simulink model "World_01_Base_Map_cs"  (R2019a)
settings: Solver=FixedStepDiscrete  StartTime=0.0  StopTime=40  FixedStep=1/300  RelTol=1e-3
PreLoadFcn:
  | mbxruntime.callbacks.PreLoadFcn(bdroot);
  | check_NUTS_defined
  | model_closed = 0;
  | assignin('base',['model_closed_' bdroot],false);
PostLoadFcn:
  | mbxruntime.callbacks.PostLoadFcn(bdroot);
InitFcn:
  | mbxruntime.callbacks.InitFcn(bdroot);
StartFcn:
  | mbxruntime.callbacks.StartFcn(bdroot);
StopFcn:
  | mbxruntime.callbacks.StopFcn(bdroot);;
  | 
model workspace: external: MAT-File .\Base_Map_Closed_cs_hws.mat (data not in the file)
undefined symbols (not defined in the file): AngularVelocity, Clock_, Data, Data_SL_Info, DiscIntNeverNeededParam, Encoding, Encoding_SL_Info, Header, Height, InitImageOutputDir, LinearAcceleration, mbxruntime, Orientation, Pose, Poses, Poses_SL_Info, Position, Step, tabledata, Twist, Width
libraries: robotlib x26, simulink_extras x22, simulink x10, PreScanSimulinkLibrary x4, dspindex x4, sharedtransform x3, robotcorelib x2, visionconversions x2, visionsinks x2
(part 1 of 7)
CloseFcn:
  | mbxruntime.callbacks.CloseFcn(bdroot);
  | evalin('base',['clear model_closed_' bdroot]);
  | model_closed = 1;
settings Model: Creator=PRESCAN  LastModifiedBy=adeye
settings DataIOCC: LimitDataPoints=on  SaveFormat=Array  SignalLoggingSaveFormat=ModelDataLogs  ReturnWorkspaceOutputs=off
settings OptimizationCC: DefaultParameterBehavior=Inlined  ExpressionDepthLimit=2147483647  InitFltsAndDblsToZero=on  LifeSpan=inf
settings DebuggingCC: SaveWithParameterizedLinksMsg=none  UnderspecifiedInitializationDetection=Classic  MergeDetectMultiDrivingBlocksExec=none  SignalResolutionControl=TryResolveAllWithWarning  MultiTaskDSMMsg=warning  MultiTaskCondExecSysMsg=none  FcnCallInpInsideContextMsg=warning  StateNameClashWarn=warning  SFUnexpectedBacktrackingDiag=warning  SFNoUnconditionalDefaultTransitionDiag=warning  SFExecutionAtInitializationDiag=none  ArithmeticOperatorsInVariantConditions=warning
settings HardwareCC: ProdBitPerPointer=32  ProdBitPerSizeT=32  ProdBitPerPtrDiffT=32  ProdLargestAtomicFloat=None  ProdIntDivRoundTo=Undefined  ProdEndianess=Unspecified  ProdWordSize=32  ProdHWDeviceType=32-bit Generic
settings ModelReferenceCC: UpdateModelReferenceTargets=IfOutOfDate  PropagateSignalLabelsOutOfModel=off
settings SFSimCC: SimUseLocalCustomCode=off  SimParseCustomCode=off
settings SFSimCC: SimCustomHeaderCode=|
  | #include "prescan.h"
  | #include "prescan_platform.h"
settings RTWCC: RTWUseLocalCustomCode=off
settings CodeAppCC: StateflowObjectComments=on
settings GRTTargetCC: TargetFcnLib=ansi_tfl_tmw.mat  TargetLangStandard=C89/C90 (ANSI)  GeneratePreprocessorConditionals=Disable all  CombineOutputUpdateFcns=off  GRTInterface=on
settings ConfigComp: CovMetricSettings=dw  CovHtmlReporting=on  CovSaveCumulativeToWorkspaceVar=on  CovSaveSingleToWorkspaceVar=on  CovExternalEMLEnable=off

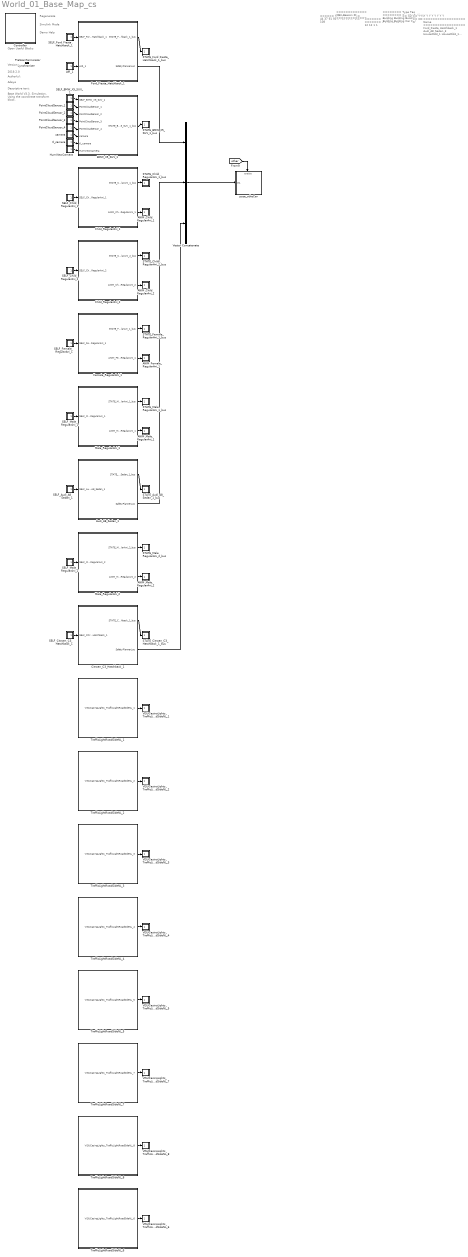
== system World_01_Base_Map_cs ==
  note: Regenerate
  note: Simulink Mode
  note: Open Useful Blocks
  note: 2019.2.0
  note: Version:
  note: Author(s):
  note: Adeye
  note: Descriptive text:
  note: Base World V3.3. Simulation,
      |
      |
      |
      | Using the coordinate transform
      | block.
  note: Demo Help
  note: ======
      | Num ID
      | ======
      | 44
      | 37
      | 91
      | 93
      | 94
      | 95
      | 96
      | 97
      | 102
      | 108
  note: =============
      | OBU-Beacon ID
      | =============
  note: =======
      | Type ID
      | =======
      | 1
      | 1
      | 12
      | 12
      | 12
      | 12
      | 12
      | 12
      | 1
      | 1
  note: ========
      | Type Tag
      | ========
      | Car
      | Car
      | Building
      | Building
      | Building
      | Building
      | Building
      | Building
      | Car
      | Car
  note: ==
      | SD
      | ==
      | Y
      | Y
      | Y
      | Y
      | Y
      | Y
      | Y
      | Y
      | Y
      | Y
  note: ==
      | CD
      | ==
      | N
      | N
      | N
      | N
      | N
      | N
      | N
      | N
      | N
      | N
  note: ==================
      | Name
      | ==================
      | Ford_Fiesta_Hatchback_1
      | Audi_A8_Sedan_3
      | HouseOld3_1
      | HouseOld4_1
      | HouseOld5_1
      | School_1
      | OfficeBrownFlat_1
      | OfficeBrownTall2_1
      | Audi_A8_Sedan_1
      | Citroen_C3_Hatchback_1
  AIR_1 : Subsystem  Tag=sensor/AIR  Priority=3  LoadFcn=load('PrescanAIRSensorData.mat');load('PrescanAIRSensorMessage.mat')  mask(PreScan Source Block: Actor Independent Receiver (AIR)){}
      mask help:
      | The Actor Information Receiver sensor provides a fast, simple and generic detection solution which is not tied up to a specific technology. The AIR detects the intersection point of the bounding box with the straight line from the sensor axis system to the middle of the bounding box.
      |
      | For more information, please click Help.
      settings: OpenFcn=open_system([gcb '/Sensor'],'mask')
      mask Help: eval('openHelp(413)')
      mask Display: image(imread('AIR.png'))
  ANIM_Child_RegularAni_1 : Subsystem  Tag=actuator/AnimationOutport  Priority=0  LoadFcn=load('PreScanAnimActuatorData.mat')  mask(PreScan Sink Block: State Animation){}
      mask help: The Human Animation port allows the human to walk, run or bend
      settings: OpenFcn=open_system([gcb '/Actuator'],'mask')
      mask Help: eval('openHelp(239)')
      mask Display: image(imread('HumanAnimated.jpg'))
  ANIM_Child_RegularAni_2 : Subsystem  Tag=actuator/AnimationOutport  Priority=0  LoadFcn=load('PreScanAnimActuatorData.mat')  mask(PreScan Sink Block: State Animation){}
      mask help: The Human Animation port allows the human to walk, run or bend
      settings: OpenFcn=open_system([gcb '/Actuator'],'mask')
      mask Help: eval('openHelp(239)')
      mask Display: image(imread('HumanAnimated.jpg'))
  ANIM_Female_RegularAni_1 : Subsystem  Tag=actuator/AnimationOutport  Priority=0  LoadFcn=load('PreScanAnimActuatorData.mat')  mask(PreScan Sink Block: State Animation){}
      mask help: The Human Animation port allows the human to walk, run or bend
      settings: OpenFcn=open_system([gcb '/Actuator'],'mask')
      mask Help: eval('openHelp(239)')
      mask Display: image(imread('HumanAnimated.jpg'))
  ANIM_Male_RegularAni_1 : Subsystem  Tag=actuator/AnimationOutport  Priority=0  LoadFcn=load('PreScanAnimActuatorData.mat')  mask(PreScan Sink Block: State Animation){}
      mask help: The Human Animation port allows the human to walk, run or bend
      settings: OpenFcn=open_system([gcb '/Actuator'],'mask')
      mask Help: eval('openHelp(239)')
      mask Display: image(imread('HumanAnimated.jpg'))
  ANIM_Male_RegularAni_2 : Subsystem  Tag=actuator/AnimationOutport  Priority=0  LoadFcn=load('PreScanAnimActuatorData.mat')  mask(PreScan Sink Block: State Animation){}
      mask help: The Human Animation port allows the human to walk, run or bend
      settings: OpenFcn=open_system([gcb '/Actuator'],'mask')
      mask Help: eval('openHelp(239)')
      mask Display: image(imread('HumanAnimated.jpg'))
  Audi_A8_Sedan_1 : Subsystem  Tag=WorldObjectSubSystem  InitFcn=UniqueId = '18645';
      mask init:
      | modelPath = GenericModelHelper.getGenericModelFilePath('ModelDepo','Vehicles\Audi_A8\Audi_A8.pgmb','e33fe1ddcf3e8ae97caccbc8f2fa74ac');imagePath = GenericModelHelper.getCompilationPicture(modelPath, 'Audi_A8_HighPoly.png');
      mask Display: image(imread(imagePath));color('white');text(0, 0, ' ID=102\n')
  BMW_X5_SUV_1 : Subsystem  Tag=WorldObjectSubSystem  InitFcn=UniqueId = '9040';
      mask init:
      | modelPath = GenericModelHelper.getGenericModelFilePath('ModelDepo','Vehicles\BMW_X5\BMW_X5.pgmb','bfeb1c11467705ab888b3011684c848b');imagePath = GenericModelHelper.getCompilationPicture(modelPath, 'BMW_X5_HighPoly.png');
      mask Display: image(imread(imagePath));color('white');text(0, 0, ' ID=55\n')
  Child_RegularAni_1 : Subsystem  Tag=WorldObjectSubSystem  InitFcn=UniqueId = '18395';
      mask init:
      | imagePath=which('Child_RegularAni.jpg');
      mask Display: image(imread(imagePath));color('white');text(0, 0, ' ID=112\n')
  Child_RegularAni_2 : Subsystem  Tag=WorldObjectSubSystem  InitFcn=UniqueId = '18628';
      mask init:
      | imagePath=which('Child_RegularAni.jpg');
      mask Display: image(imread(imagePath));color('white');text(0, 0, ' ID=111\n')
  Citroen_C3_Hatchback_1 : Subsystem  Tag=WorldObjectSubSystem  InitFcn=UniqueId = '18857';
      mask init:
      | modelPath = GenericModelHelper.getGenericModelFilePath('ModelDepo','Vehicles\Citroen_C3\Citroen_C3.pgmb','e804ced06d50dbfc6a2202ab3ad01b0c');imagePath = GenericModelHelper.getCompilationPicture(modelPath, 'Citroen_C3_HighPoly.png');
      mask Display: image(imread(imagePath));color('white');text(0, 0, ' ID=108\n')
  Controller : Subsystem  Description=8A3CD2955739A82C886C20AE3E253D78460D53180EE2C1B14CC08DF75A70BE77  Priority=-1  LoadFcn=load PreScanControllerData  mask(PreScan Simulation Controller){prescanversion='2019.2.0', ModelReferencing=off, TimeStep=1/300, ControlMode=0, PreScanExecutionMode=on, ControllerCount=0, ControllerIndex=0, ControllerOptions=''}
      mask prompts: prescanversion "PreScan Version"; ModelReferencing "Use Model Referencing"; TimeStep "Upload Period [s]"; ControlMode "Control Mode"; PreScanExecutionMode "Execution Mode"; ControllerCount "Controller Count"; ControllerIndex "Controller Index"; ControllerOptions "Controller Options"
      mask help:
      | Please do not remove this block from the compilation sheet,
      | as it connects the model to the PreScan environment.
      mask init:
      | model = bdroot(gcb);
      | ExperimentFile = mbxruntime.findExperimentFile(model,true); %relative path
      | 
      | [d1, d2, d3, prescandata] = prescan_Settings();
      | ModelDepo = fullfile(prescandata,'ModelDepo'); 
      | 
      | RTmode = mbxruntime.getRTMode(model);
      | 
      | SimulationMode = get_param(bdroot,'SimulationMode');
      | if strcmp(SimulationMode, 'rapid-accelerator')
      |     SimulationMode = 'external';
      | end
      | TargetName = get_param(bdroot,'SystemTargetFile');
      settings: ModelCloseFcn=assignin('base',['model_closed_' bdroot],true);
      mask Help: eval('openHelp(812)')
      mask Display: image(imread('prescanlogo.ico'))
  Female_RegularAni_1 : Subsystem  Tag=WorldObjectSubSystem  InitFcn=UniqueId = '18631';
      mask init:
      | imagePath=which('Female_RegularAni.jpg');
      mask Display: image(imread(imagePath));color('white');text(0, 0, ' ID=113\n')
  Ford_Fiesta_Hatchback_1 : Subsystem  Tag=WorldObjectSubSystem  InitFcn=UniqueId = '4876';
      mask init:
      | modelPath = GenericModelHelper.getGenericModelFilePath('ModelDepo','Vehicles\Ford_Fiesta\Ford_Fiesta.pgmb','fe2c7a73e0a60cba76689b71cd1bb76a');imagePath = GenericModelHelper.getCompilationPicture(modelPath, 'Ford_Fiesta_HighPoly.png');
      mask Display: image(imread(imagePath));color('white');text(0, 0, ' ID=44\n')
  HumViewCamera : Subsystem  Tag=sensor/Camera/CameraSensor  Priority=3  mask(PreScan Source Block: Camera Sensor){}
      mask help: The Camera Sensor provides a color or monochrome image.
      settings: OpenFcn=open_system([gcb '/Sensor'],'mask')
      mask Help: eval('openHelp(457)')
      mask Display: image(imread('CameraSensor.png'))
  Male_RegularAni_1 : Subsystem  Tag=WorldObjectSubSystem  InitFcn=UniqueId = '18634';
      mask init:
      | imagePath=which('Male_RegularAni.jpg');
      mask Display: image(imread(imagePath));color('white');text(0, 0, ' ID=114\n')
  Male_RegularAni_2 : Subsystem  Tag=WorldObjectSubSystem  InitFcn=UniqueId = '18853';
      mask init:
      | imagePath=which('Male_RegularAni.jpg');
      mask Display: image(imread(imagePath));color('white');text(0, 0, ' ID=107\n')
  PointCloudSensor_1 : Subsystem  Tag=sensor/PointCloudInport  Priority=3  mask(PreScan Source Block: Point Cloud Sensor){}
      mask help: The Point Cloud Sensor provides XYZ positions relative to the sensor
      settings: OpenFcn=open_system([gcb '/Sensor'],'mask')
      mask Help: eval('openHelp(6400)')
      mask Display: image(imread('PointCloudSensorSL.png'))
  PointCloudSensor_2 : Subsystem  Tag=sensor/PointCloudInport  Priority=3  mask(PreScan Source Block: Point Cloud Sensor){}
      mask help: The Point Cloud Sensor provides XYZ positions relative to the sensor
      settings: OpenFcn=open_system([gcb '/Sensor'],'mask')
      mask Help: eval('openHelp(6400)')
      mask Display: image(imread('PointCloudSensorSL.png'))
  PointCloudSensor_3 : Subsystem  Tag=sensor/PointCloudInport  Priority=3  mask(PreScan Source Block: Point Cloud Sensor){}
      mask help: The Point Cloud Sensor provides XYZ positions relative to the sensor
      settings: OpenFcn=open_system([gcb '/Sensor'],'mask')
      mask Help: eval('openHelp(6400)')
      mask Display: image(imread('PointCloudSensorSL.png'))
  PointCloudSensor_4 : Subsystem  Tag=sensor/PointCloudInport  Priority=3  mask(PreScan Source Block: Point Cloud Sensor){}
      mask help: The Point Cloud Sensor provides XYZ positions relative to the sensor
      settings: OpenFcn=open_system([gcb '/Sensor'],'mask')
      mask Help: eval('openHelp(6400)')
      mask Display: image(imread('PointCloudSensorSL.png'))
  PreScanTerminator : Subsystem  Tag=PreScanTerminator  Priority=999  LoadFcn=load PrescanTerminatorData  mask(PreScan Simulation Terminator){TimeStep=1/300}
      mask prompts: TimeStep "Upload Period [s]"
      mask help:
      | Please do not remove this block from the compilation sheet as it
      | connects the model to the PreScan environment.
      mask Help: eval('openHelp(812)')
      mask Display: image(imread('prescanlogo.ico'))
  SELF_Audi_A8_Sedan_1 : Subsystem  Tag=sensor/SelfPort  Priority=3  LoadFcn=load('PreScanSelfSensorData.mat')  mask(PreScan Source Block: SELF){}
      mask help:
      | The SELF port shows (state) information of the actor itself. The outputs are position in the experiment's axis system and the GPS coordinates, and the object's absolute velocity and compass heading.
      |
      | For more information, please click Help.
      settings: OpenFcn=open_system([gcb '/Sensor'],'mask')
      mask Help: eval('openHelp(462)')
      mask Display: image(imread('GPS.png'))
  SELF_BMW_X5_SUV_1 : Subsystem  Tag=sensor/SelfPort  Priority=3  LoadFcn=load('PreScanSelfSensorData.mat')  mask(PreScan Source Block: SELF){}
      mask help:
      | The SELF port shows (state) information of the actor itself. The outputs are position in the experiment's axis system and the GPS coordinates, and the object's absolute velocity and compass heading.
      |
      | For more information, please click Help.
      settings: OpenFcn=open_system([gcb '/Sensor'],'mask')
      mask Help: eval('openHelp(462)')
      mask Display: image(imread('GPS.png'))
  SELF_Child_RegularAni_1 : Subsystem  Tag=sensor/SelfPort  Priority=3  LoadFcn=load('PreScanSelfSensorData.mat')  mask(PreScan Source Block: SELF){}
      mask help:
      | The SELF port shows (state) information of the actor itself. The outputs are position in the experiment's axis system and the GPS coordinates, and the object's absolute velocity and compass heading.
      |
      | For more information, please click Help.
      settings: OpenFcn=open_system([gcb '/Sensor'],'mask')
      mask Help: eval('openHelp(462)')
      mask Display: image(imread('GPS.png'))
  SELF_Child_RegularAni_2 : Subsystem  Tag=sensor/SelfPort  Priority=3  LoadFcn=load('PreScanSelfSensorData.mat')  mask(PreScan Source Block: SELF){}
      mask help:
      | The SELF port shows (state) information of the actor itself. The outputs are position in the experiment's axis system and the GPS coordinates, and the object's absolute velocity and compass heading.
      |
      | For more information, please click Help.
      settings: OpenFcn=open_system([gcb '/Sensor'],'mask')
      mask Help: eval('openHelp(462)')
      mask Display: image(imread('GPS.png'))
  SELF_Citroen_C3_Hatchback_1 : Subsystem  Tag=sensor/SelfPort  Priority=3  LoadFcn=load('PreScanSelfSensorData.mat')  mask(PreScan Source Block: SELF){}
      mask help:
      | The SELF port shows (state) information of the actor itself. The outputs are position in the experiment's axis system and the GPS coordinates, and the object's absolute velocity and compass heading.
      |
      | For more information, please click Help.
      settings: OpenFcn=open_system([gcb '/Sensor'],'mask')
      mask Help: eval('openHelp(462)')
      mask Display: image(imread('GPS.png'))
  SELF_Female_RegularAni_1 : Subsystem  Tag=sensor/SelfPort  Priority=3  LoadFcn=load('PreScanSelfSensorData.mat')  mask(PreScan Source Block: SELF){}
      mask help:
      | The SELF port shows (state) information of the actor itself. The outputs are position in the experiment's axis system and the GPS coordinates, and the object's absolute velocity and compass heading.
      |
      | For more information, please click Help.
      settings: OpenFcn=open_system([gcb '/Sensor'],'mask')
      mask Help: eval('openHelp(462)')
      mask Display: image(imread('GPS.png'))
  SELF_Ford_Fiesta_Hatchback_1 : Subsystem  Tag=sensor/SelfPort  Priority=3  LoadFcn=load('PreScanSelfSensorData.mat')  mask(PreScan Source Block: SELF){}
      mask help:
      | The SELF port shows (state) information of the actor itself. The outputs are position in the experiment's axis system and the GPS coordinates, and the object's absolute velocity and compass heading.
      |
      | For more information, please click Help.
      settings: OpenFcn=open_system([gcb '/Sensor'],'mask')
      mask Help: eval('openHelp(462)')
      mask Display: image(imread('GPS.png'))
  SELF_Male_RegularAni_1 : Subsystem  Tag=sensor/SelfPort  Priority=3  LoadFcn=load('PreScanSelfSensorData.mat')  mask(PreScan Source Block: SELF){}
      mask help:
      | The SELF port shows (state) information of the actor itself. The outputs are position in the experiment's axis system and the GPS coordinates, and the object's absolute velocity and compass heading.
      |
      | For more information, please click Help.
      settings: OpenFcn=open_system([gcb '/Sensor'],'mask')
      mask Help: eval('openHelp(462)')
      mask Display: image(imread('GPS.png'))
  SELF_Male_RegularAni_2 : Subsystem  Tag=sensor/SelfPort  Priority=3  LoadFcn=load('PreScanSelfSensorData.mat')  mask(PreScan Source Block: SELF){}
      mask help:
      | The SELF port shows (state) information of the actor itself. The outputs are position in the experiment's axis system and the GPS coordinates, and the object's absolute velocity and compass heading.
      |
      | For more information, please click Help.
      settings: OpenFcn=open_system([gcb '/Sensor'],'mask')
      mask Help: eval('openHelp(462)')
      mask Display: image(imread('GPS.png'))
  STATE_Audi_A8_Sedan_1_bus : Subsystem  Tag=actuator/StatePort  Priority=0  LoadFcn=load('PreScanStateActuatorData.mat')  mask(PreScan Sink Block: State){}
      mask help:
      | The Actor State contains a vector signal of size (9x1), containing the following signals:
      |
      | -  Position    	(x,y,z)             	[m]
      | -  Velocity    	(vx,vy,vz)         	[m/s]
      | -  Angles       	(Roll, Pitch, Yaw)	[rad]
      |
      | The Actor state is defined in the global axis system.
      | The state is superponed on the Initial position defined in the GUI.
      |
      | For more information, please click Help.
      settings: OpenFcn=open_system([gcb '/Actuator'],'mask')
      mask Help: eval('openHelp(222)')
      mask Display: image(imread('State.png'))
  STATE_BMW_X5_SUV_1_bus : Subsystem  Tag=actuator/StatePort  Priority=0  LoadFcn=load('PreScanStateActuatorData.mat')  mask(PreScan Sink Block: State){}
      mask help:
      | The Actor State contains a vector signal of size (9x1), containing the following signals:
      |
      | -  Position    	(x,y,z)             	[m]
      | -  Velocity    	(vx,vy,vz)         	[m/s]
      | -  Angles       	(Roll, Pitch, Yaw)	[rad]
      |
      | The Actor state is defined in the global axis system.
      | The state is superponed on the Initial position defined in the GUI.
      |
      | For more information, please click Help.
      settings: OpenFcn=open_system([gcb '/Actuator'],'mask')
      mask Help: eval('openHelp(222)')
      mask Display: image(imread('State.png'))
  STATE_Child_RegularAni_1_bus : Subsystem  Tag=actuator/StatePort  Priority=0  LoadFcn=load('PreScanStateActuatorData.mat')  mask(PreScan Sink Block: State){}
      mask help:
      | The Actor State contains a vector signal of size (9x1), containing the following signals:
      |
      | -  Position    	(x,y,z)             	[m]
      | -  Velocity    	(vx,vy,vz)         	[m/s]
      | -  Angles       	(Roll, Pitch, Yaw)	[rad]
      |
      | The Actor state is defined in the global axis system.
      | The state is superponed on the Initial position defined in the GUI.
      |
      | For more information, please click Help.
      settings: OpenFcn=open_system([gcb '/Actuator'],'mask')
      mask Help: eval('openHelp(222)')
      mask Display: image(imread('State.png'))
  STATE_Child_RegularAni_2_bus : Subsystem  Tag=actuator/StatePort  Priority=0  LoadFcn=load('PreScanStateActuatorData.mat')  mask(PreScan Sink Block: State){}
      mask help:
      | The Actor State contains a vector signal of size (9x1), containing the following signals:
      |
      | -  Position    	(x,y,z)             	[m]
      | -  Velocity    	(vx,vy,vz)         	[m/s]
      | -  Angles       	(Roll, Pitch, Yaw)	[rad]
      |
      | The Actor state is defined in the global axis system.
      | The state is superponed on the Initial position defined in the GUI.
      |
      | For more information, please click Help.
      settings: OpenFcn=open_system([gcb '/Actuator'],'mask')
      mask Help: eval('openHelp(222)')
      mask Display: image(imread('State.png'))
  STATE_Citroen_C3_Hatchback_1_bus : Subsystem  Tag=actuator/StatePort  Priority=0  LoadFcn=load('PreScanStateActuatorData.mat')  mask(PreScan Sink Block: State){}
      mask help:
      | The Actor State contains a vector signal of size (9x1), containing the following signals:
      |
      | -  Position    	(x,y,z)             	[m]
      | -  Velocity    	(vx,vy,vz)         	[m/s]
      | -  Angles       	(Roll, Pitch, Yaw)	[rad]
      |
      | The Actor state is defined in the global axis system.
      | The state is superponed on the Initial position defined in the GUI.
      |
      | For more information, please click Help.
      settings: OpenFcn=open_system([gcb '/Actuator'],'mask')
      mask Help: eval('openHelp(222)')
      mask Display: image(imread('State.png'))
  STATE_Female_RegularAni_1_bus : Subsystem  Tag=actuator/StatePort  Priority=0  LoadFcn=load('PreScanStateActuatorData.mat')  mask(PreScan Sink Block: State){}
      mask help:
      | The Actor State contains a vector signal of size (9x1), containing the following signals:
      |
      | -  Position    	(x,y,z)             	[m]
      | -  Velocity    	(vx,vy,vz)         	[m/s]
      | -  Angles       	(Roll, Pitch, Yaw)	[rad]
      |
      | The Actor state is defined in the global axis system.
      | The state is superponed on the Initial position defined in the GUI.
      |
      | For more information, please click Help.
      settings: OpenFcn=open_system([gcb '/Actuator'],'mask')
      mask Help: eval('openHelp(222)')
      mask Display: image(imread('State.png'))
  STATE_Ford_Fiesta_Hatchback_1_bus : Subsystem  Tag=actuator/StatePort  Priority=0  LoadFcn=load('PreScanStateActuatorData.mat')  mask(PreScan Sink Block: State){}
      mask help:
      | The Actor State contains a vector signal of size (9x1), containing the following signals:
      |
      | -  Position    	(x,y,z)             	[m]
      | -  Velocity    	(vx,vy,vz)         	[m/s]
      | -  Angles       	(Roll, Pitch, Yaw)	[rad]
      |
      | The Actor state is defined in the global axis system.
      | The state is superponed on the Initial position defined in the GUI.
      |
      | For more information, please click Help.
      settings: OpenFcn=open_system([gcb '/Actuator'],'mask')
      mask Help: eval('openHelp(222)')
      mask Display: image(imread('State.png'))
  STATE_Male_RegularAni_1_bus : Subsystem  Tag=actuator/StatePort  Priority=0  LoadFcn=load('PreScanStateActuatorData.mat')  mask(PreScan Sink Block: State){}
      mask help:
      | The Actor State contains a vector signal of size (9x1), containing the following signals:
      |
      | -  Position    	(x,y,z)             	[m]
      | -  Velocity    	(vx,vy,vz)         	[m/s]
      | -  Angles       	(Roll, Pitch, Yaw)	[rad]
      |
      | The Actor state is defined in the global axis system.
      | The state is superponed on the Initial position defined in the GUI.
      |
      | For more information, please click Help.
      settings: OpenFcn=open_system([gcb '/Actuator'],'mask')
      mask Help: eval('openHelp(222)')
      mask Display: image(imread('State.png'))
  STATE_Male_RegularAni_2_bus : Subsystem  Tag=actuator/StatePort  Priority=0  LoadFcn=load('PreScanStateActuatorData.mat')  mask(PreScan Sink Block: State){}
      mask help:
      | The Actor State contains a vector signal of size (9x1), containing the following signals:
      |
      | -  Position    	(x,y,z)             	[m]
      | -  Velocity    	(vx,vy,vz)         	[m/s]
      | -  Angles       	(Roll, Pitch, Yaw)	[rad]
      |
      | The Actor state is defined in the global axis system.
      | The state is superponed on the Initial position defined in the GUI.
      |
      | For more information, please click Help.
      settings: OpenFcn=open_system([gcb '/Actuator'],'mask')
      mask Help: eval('openHelp(222)')
      mask Display: image(imread('State.png'))
  Synchronizer : Subsystem  Tag=PreScanSynchronizer  Priority=1  LoadFcn=load PrescanSynchronizeData  mask(PreScan Simulation Core Block){TimeStep=1/300}
      mask prompts: TimeStep "Timestep [s]"
      mask help:
      | Please do not remove this block from the PreScan compilation sheet,
      | as it contains essential configuration parameters for a PreScan simulation.
      settings: DeleteFcn=PreScanBlockDeleteFcn;
      mask Display: image(imread('prescanlogo.ico'))
  TrafficLightRoadSideNL_1 : Subsystem  Tag=WorldObjectSubSystem  InitFcn=UniqueId = '646';
      mask init:
      | imagePath=which('TrafficLightRoadSideNL.jpg');
      mask Display: image(imread(imagePath));color('white');text(0, 0, ' ID=76\n')
  TrafficLightRoadSideNL_2 : Subsystem  Tag=WorldObjectSubSystem  InitFcn=UniqueId = '647';
      mask init:
      | imagePath=which('TrafficLightRoadSideNL.jpg');
      mask Display: image(imread(imagePath));color('white');text(0, 0, ' ID=77\n')
  TrafficLightRoadSideNL_3 : Subsystem  Tag=WorldObjectSubSystem  InitFcn=UniqueId = '649';
      mask init:
      | imagePath=which('TrafficLightRoadSideNL.jpg');
      mask Display: image(imread(imagePath));color('white');text(0, 0, ' ID=78\n')
  TrafficLightRoadSideNL_4 : Subsystem  Tag=WorldObjectSubSystem  InitFcn=UniqueId = '650';
      mask init:
      | imagePath=which('TrafficLightRoadSideNL.jpg');
      mask Display: image(imread(imagePath));color('white');text(0, 0, ' ID=79\n')
  TrafficLightRoadSideNL_5 : Subsystem  Tag=WorldObjectSubSystem  InitFcn=UniqueId = '651';
      mask init:
      | imagePath=which('TrafficLightRoadSideNL.jpg');
      mask Display: image(imread(imagePath));color('white');text(0, 0, ' ID=80\n')
  TrafficLightRoadSideNL_6 : Subsystem  Tag=WorldObjectSubSystem  InitFcn=UniqueId = '10446';
      mask init:
      | imagePath=which('TrafficLightRoadSideNL.jpg');
      mask Display: image(imread(imagePath));color('white');text(0, 0, ' ID=81\n')
  TrafficLightRoadSideNL_7 : Subsystem  Tag=WorldObjectSubSystem  InitFcn=UniqueId = '653';
      mask init:
      | imagePath=which('TrafficLightRoadSideNL.jpg');
      mask Display: image(imread(imagePath));color('white');text(0, 0, ' ID=82\n')
  TrafficLightRoadSideNL_8 : Subsystem  Tag=WorldObjectSubSystem  InitFcn=UniqueId = '654';
      mask init:
      | imagePath=which('TrafficLightRoadSideNL.jpg');
      mask Display: image(imread(imagePath));color('white');text(0, 0, ' ID=83\n')
  VISUCasingLights_TrafficLightRoadSideNL_1 : Subsystem  Tag=actuator/VisuCasingLights  Priority=0  mask(PreScan Sink Block: VisuTrafficLight){UniqueID=646, ColorsObjectQuery=, Colors=[]}
      mask prompts: UniqueID "Parent Unique Identifier"; ColorsObjectQuery "Query for Color Object"; Colors "Matrix of colors"
      mask help:
      | The VisuTrafficLight block provides a way to animate traffic lights: switch on and off individual lights.
      |
      | For more information, please click Help.
      settings: OpenFcn=open_system([gcb '/Actuator'],'mask')
      mask Help: eval('openHelp(731)')
      mask Display: image(imread('TrafficLightCasing.png'))
  VISUCasingLights_TrafficLightRoadSideNL_2 : Subsystem  Tag=actuator/VisuCasingLights  Priority=0  mask(PreScan Sink Block: VisuTrafficLight){UniqueID=647, ColorsObjectQuery=, Colors=[]}
      mask prompts: UniqueID "Parent Unique Identifier"; ColorsObjectQuery "Query for Color Object"; Colors "Matrix of colors"
      mask help:
      | The VisuTrafficLight block provides a way to animate traffic lights: switch on and off individual lights.
      |
      | For more information, please click Help.
      settings: OpenFcn=open_system([gcb '/Actuator'],'mask')
      mask Help: eval('openHelp(731)')
      mask Display: image(imread('TrafficLightCasing.png'))
  VISUCasingLights_TrafficLightRoadSideNL_3 : Subsystem  Tag=actuator/VisuCasingLights  Priority=0  mask(PreScan Sink Block: VisuTrafficLight){UniqueID=649, ColorsObjectQuery=, Colors=[]}
      mask prompts: UniqueID "Parent Unique Identifier"; ColorsObjectQuery "Query for Color Object"; Colors "Matrix of colors"
      mask help:
      | The VisuTrafficLight block provides a way to animate traffic lights: switch on and off individual lights.
      |
      | For more information, please click Help.
      settings: OpenFcn=open_system([gcb '/Actuator'],'mask')
      mask Help: eval('openHelp(731)')
      mask Display: image(imread('TrafficLightCasing.png'))
  VISUCasingLights_TrafficLightRoadSideNL_4 : Subsystem  Tag=actuator/VisuCasingLights  Priority=0  mask(PreScan Sink Block: VisuTrafficLight){UniqueID=650, ColorsObjectQuery=, Colors=[]}
      mask prompts: UniqueID "Parent Unique Identifier"; ColorsObjectQuery "Query for Color Object"; Colors "Matrix of colors"
      mask help:
      | The VisuTrafficLight block provides a way to animate traffic lights: switch on and off individual lights.
      |
      | For more information, please click Help.
      settings: OpenFcn=open_system([gcb '/Actuator'],'mask')
      mask Help: eval('openHelp(731)')
      mask Display: image(imread('TrafficLightCasing.png'))
  VISUCasingLights_TrafficLightRoadSideNL_5 : Subsystem  Tag=actuator/VisuCasingLights  Priority=0  mask(PreScan Sink Block: VisuTrafficLight){UniqueID=651, ColorsObjectQuery=, Colors=[]}
      mask prompts: UniqueID "Parent Unique Identifier"; ColorsObjectQuery "Query for Color Object"; Colors "Matrix of colors"
      mask help:
      | The VisuTrafficLight block provides a way to animate traffic lights: switch on and off individual lights.
      |
      | For more information, please click Help.
      settings: OpenFcn=open_system([gcb '/Actuator'],'mask')
      mask Help: eval('openHelp(731)')
      mask Display: image(imread('TrafficLightCasing.png'))
  VISUCasingLights_TrafficLightRoadSideNL_6 : Subsystem  Tag=actuator/VisuCasingLights  Priority=0  mask(PreScan Sink Block: VisuTrafficLight){UniqueID=10446, ColorsObjectQuery=, Colors=[]}
      mask prompts: UniqueID "Parent Unique Identifier"; ColorsObjectQuery "Query for Color Object"; Colors "Matrix of colors"
      mask help:
      | The VisuTrafficLight block provides a way to animate traffic lights: switch on and off individual lights.
      |
      | For more information, please click Help.
      settings: OpenFcn=open_system([gcb '/Actuator'],'mask')
      mask Help: eval('openHelp(731)')
      mask Display: image(imread('TrafficLightCasing.png'))
  VISUCasingLights_TrafficLightRoadSideNL_7 : Subsystem  Tag=actuator/VisuCasingLights  Priority=0  mask(PreScan Sink Block: VisuTrafficLight){UniqueID=653, ColorsObjectQuery=, Colors=[]}
      mask prompts: UniqueID "Parent Unique Identifier"; ColorsObjectQuery "Query for Color Object"; Colors "Matrix of colors"
      mask help:
      | The VisuTrafficLight block provides a way to animate traffic lights: switch on and off individual lights.
      |
      | For more information, please click Help.
      settings: OpenFcn=open_system([gcb '/Actuator'],'mask')
      mask Help: eval('openHelp(731)')
      mask Display: image(imread('TrafficLightCasing.png'))
  VISUCasingLights_TrafficLightRoadSideNL_8 : Subsystem  Tag=actuator/VisuCasingLights  Priority=0  mask(PreScan Sink Block: VisuTrafficLight){UniqueID=654, ColorsObjectQuery=, Colors=[]}
      mask prompts: UniqueID "Parent Unique Identifier"; ColorsObjectQuery "Query for Color Object"; Colors "Matrix of colors"
      mask help:
      | The VisuTrafficLight block provides a way to animate traffic lights: switch on and off individual lights.
      |
      | For more information, please click Help.
      settings: OpenFcn=open_system([gcb '/Actuator'],'mask')
      mask Help: eval('openHelp(731)')
      mask Display: image(imread('TrafficLightCasing.png'))
  Vector Concatenate : Concatenate  NumInputs=3
  camera : Subsystem  Tag=sensor/Camera/CameraSensor  Priority=3  mask(PreScan Source Block: Camera Sensor){}
      mask help: The Camera Sensor provides a color or monochrome image.
      settings: OpenFcn=open_system([gcb '/Sensor'],'mask')
      mask Help: eval('openHelp(457)')
      mask Display: image(imread('CameraSensor.png'))
  pose_otheCar : Subsystem
  tl_camera : Subsystem  Tag=sensor/Camera/CameraSensor  Priority=3  mask(PreScan Source Block: Camera Sensor){}
      mask help: The Camera Sensor provides a color or monochrome image.
      settings: OpenFcn=open_system([gcb '/Sensor'],'mask')
      mask Help: eval('openHelp(457)')
      mask Display: image(imread('CameraSensor.png'))
  wires:
  [other] -> pose_otheCar/Enable
  Vector Concatenate/1 -> pose_otheCar/1(In1)
  Ford_Fiesta_Hatchback_1/2(SafetyPlannerLoc) -> Vector Concatenate/1
  Audi_A8_Sedan_1/2(SafetyPlannerLoc) -> Vector Concatenate/2
  Citroen_C3_Hatchback_1/2(SafetyPlannerLoc) -> Vector Concatenate/3
  Ford_Fiesta_Hatchback_1/1(STATE_Ford_Fiesta_Hatchback_1_bus) -> STATE_Ford_Fiesta_Hatchback_1_bus/1(STATE_Ford_Fiesta_Hatchback_1_bus)
  SELF_Ford_Fiesta_Hatchback_1/1(SELF_Ford_Fiesta_Hatchback_1) -> Ford_Fiesta_Hatchback_1/1(SELF_Ford_Fiesta_Hatchback_1)
  AIR_1/1(AIR_1) -> Ford_Fiesta_Hatchback_1/2(AIR_1)
  BMW_X5_SUV_1/1(STATE_BMW_X5_SUV_1_bus) -> STATE_BMW_X5_SUV_1_bus/1(STATE_BMW_X5_SUV_1_bus)
  SELF_BMW_X5_SUV_1/1(SELF_BMW_X5_SUV_1) -> BMW_X5_SUV_1/1(SELF_BMW_X5_SUV_1)
  PointCloudSensor_1/1(PointCloudSensor_1) -> BMW_X5_SUV_1/2(PointCloudSensor_1)
  PointCloudSensor_2/1(PointCloudSensor_2) -> BMW_X5_SUV_1/3(PointCloudSensor_2)
  PointCloudSensor_3/1(PointCloudSensor_3) -> BMW_X5_SUV_1/4(PointCloudSensor_3)
  PointCloudSensor_4/1(PointCloudSensor_4) -> BMW_X5_SUV_1/5(PointCloudSensor_4)
  camera/1(camera) -> BMW_X5_SUV_1/6(camera)
  tl_camera/1(tl_camera) -> BMW_X5_SUV_1/7(tl_camera)
  HumViewCamera/1(HumViewCamera) -> BMW_X5_SUV_1/8(HumViewCamera)
  Child_RegularAni_1/1(STATE_Child_RegularAni_1_bus) -> STATE_Child_RegularAni_1_bus/1(STATE_Child_RegularAni_1_bus)
  Child_RegularAni_1/2(ANIM_Child_RegularAni_1) -> ANIM_Child_RegularAni_1/1(ANIM_Child_RegularAni_1)
  SELF_Child_RegularAni_1/1(SELF_Child_RegularAni_1) -> Child_RegularAni_1/1(SELF_Child_RegularAni_1)
  Child_RegularAni_2/1(STATE_Child_RegularAni_2_bus) -> STATE_Child_RegularAni_2_bus/1(STATE_Child_RegularAni_2_bus)
  Child_RegularAni_2/2(ANIM_Child_RegularAni_2) -> ANIM_Child_RegularAni_2/1(ANIM_Child_RegularAni_2)
  SELF_Child_RegularAni_2/1(SELF_Child_RegularAni_2) -> Child_RegularAni_2/1(SELF_Child_RegularAni_2)
  Female_RegularAni_1/1(STATE_Female_RegularAni_1_bus) -> STATE_Female_RegularAni_1_bus/1(STATE_Female_RegularAni_1_bus)
  Female_RegularAni_1/2(ANIM_Female_RegularAni_1) -> ANIM_Female_RegularAni_1/1(ANIM_Female_RegularAni_1)
  SELF_Female_RegularAni_1/1(SELF_Female_RegularAni_1) -> Female_RegularAni_1/1(SELF_Female_RegularAni_1)
  Male_RegularAni_1/1(STATE_Male_RegularAni_1_bus) -> STATE_Male_RegularAni_1_bus/1(STATE_Male_RegularAni_1_bus)
  Male_RegularAni_1/2(ANIM_Male_RegularAni_1) -> ANIM_Male_RegularAni_1/1(ANIM_Male_RegularAni_1)
  SELF_Male_RegularAni_1/1(SELF_Male_RegularAni_1) -> Male_RegularAni_1/1(SELF_Male_RegularAni_1)
  Audi_A8_Sedan_1/1(STATE_Audi_A8_Sedan_1_bus) -> STATE_Audi_A8_Sedan_1_bus/1(STATE_Audi_A8_Sedan_1_bus)
  SELF_Audi_A8_Sedan_1/1(SELF_Audi_A8_Sedan_1) -> Audi_A8_Sedan_1/1(SELF_Audi_A8_Sedan_1)
  Male_RegularAni_2/1(STATE_Male_RegularAni_2_bus) -> STATE_Male_RegularAni_2_bus/1(STATE_Male_RegularAni_2_bus)
  Male_RegularAni_2/2(ANIM_Male_RegularAni_2) -> ANIM_Male_RegularAni_2/1(ANIM_Male_RegularAni_2)
  SELF_Male_RegularAni_2/1(SELF_Male_RegularAni_2) -> Male_RegularAni_2/1(SELF_Male_RegularAni_2)
  Citroen_C3_Hatchback_1/1(STATE_Citroen_C3_Hatchback_1_bus) -> STATE_Citroen_C3_Hatchback_1_bus/1(STATE_Citroen_C3_Hatchback_1_bus)
  SELF_Citroen_C3_Hatchback_1/1(SELF_Citroen_C3_Hatchback_1) -> Citroen_C3_Hatchback_1/1(SELF_Citroen_C3_Hatchback_1)
  TrafficLightRoadSideNL_1/1(VISUCasingLights_TrafficLightRoadSideNL_1) -> VISUCasingLights_TrafficLightRoadSideNL_1/1(VISUCasingLights_TrafficLightRoadSideNL_1)
  TrafficLightRoadSideNL_2/1(VISUCasingLights_TrafficLightRoadSideNL_2) -> VISUCasingLights_TrafficLightRoadSideNL_2/1(VISUCasingLights_TrafficLightRoadSideNL_2)
  TrafficLightRoadSideNL_3/1(VISUCasingLights_TrafficLightRoadSideNL_3) -> VISUCasingLights_TrafficLightRoadSideNL_3/1(VISUCasingLights_TrafficLightRoadSideNL_3)
  TrafficLightRoadSideNL_4/1(VISUCasingLights_TrafficLightRoadSideNL_4) -> VISUCasingLights_TrafficLightRoadSideNL_4/1(VISUCasingLights_TrafficLightRoadSideNL_4)
  TrafficLightRoadSideNL_5/1(VISUCasingLights_TrafficLightRoadSideNL_5) -> VISUCasingLights_TrafficLightRoadSideNL_5/1(VISUCasingLights_TrafficLightRoadSideNL_5)
  TrafficLightRoadSideNL_7/1(VISUCasingLights_TrafficLightRoadSideNL_7) -> VISUCasingLights_TrafficLightRoadSideNL_7/1(VISUCasingLights_TrafficLightRoadSideNL_7)
  TrafficLightRoadSideNL_8/1(VISUCasingLights_TrafficLightRoadSideNL_8) -> VISUCasingLights_TrafficLightRoadSideNL_8/1(VISUCasingLights_TrafficLightRoadSideNL_8)
  TrafficLightRoadSideNL_6/1(VISUCasingLights_TrafficLightRoadSideNL_6) -> VISUCasingLights_TrafficLightRoadSideNL_6/1(VISUCasingLights_TrafficLightRoadSideNL_6)

== system World_01_Base_Map_cs/AIR_1 ==
  Sensor : S-Function  FunctionName=sfun_AIRSensor  Parameters=detectableObjects, sensorID, timestep  SFunctionDeploymentMode=off  EnableBusSupport=off  mask(PreScan Source Block: Actor Independent Receiver (AIR)){detectableObjects=1, sensorID=4878, timestep=1/300}
      mask prompts: detectableObjects "Max detectable objects"; sensorID "Sensor ID"; timestep "MATLAB timestep:"
      mask help:
      | The Actor Information Receiver sensor provides a fast, simple and generic detection solution which is not tied up to a specific technology. The AIR detects the intersection point of the bounding box with the straight line from the sensor axis system to the middle of the bounding box.
      |
      | For more information, please click Help.
      mask Help: eval('openHelp(413)')
      mask Display: image(imread('AIR.png'))
  AIR_1 : Outport  Tag=outport/AIR  OutDataTypeStr=Bus: PRESCAN_AIRSENSORMESSAGE  PortDimensions=1  SampleTime=1/300
  wires:
  Sensor/1 -> AIR_1/1

== system World_01_Base_Map_cs/ANIM_Child_RegularAni_1 ==
  ANIM_Child_RegularAni_1 : Inport  Tag=inport/AnimationOutport  OutDataTypeStr=Bus: PRESCAN_ANIMACTUATORDATA  PortDimensions=1  SampleTime=1/300  BusOutputAsStruct=on
  Actuator : S-Function  FunctionName=sfun_AnimActuator  Parameters=UniqueID, TimeStep  SFunctionDeploymentMode=off  EnableBusSupport=off  mask(PreScan Sink Block: State Animation){UniqueID=18395, TimeStep=1/300}
      mask prompts: UniqueID "Auto-Assigned: Unique ID"; TimeStep "Auto-Assigned: Upload Period [s]"
      mask help: The Human Animation port allows the human to walk, run or bend
      mask Help: eval('openHelp(239)')
      mask Display: image(imread('HumanAnimated.jpg'))
  wires:
  ANIM_Child_RegularAni_1/1 -> Actuator/1

== system World_01_Base_Map_cs/ANIM_Child_RegularAni_2 ==
  ANIM_Child_RegularAni_2 : Inport  Tag=inport/AnimationOutport  OutDataTypeStr=Bus: PRESCAN_ANIMACTUATORDATA  PortDimensions=1  SampleTime=1/300  BusOutputAsStruct=on
  Actuator : S-Function  FunctionName=sfun_AnimActuator  Parameters=UniqueID, TimeStep  SFunctionDeploymentMode=off  EnableBusSupport=off  mask(PreScan Sink Block: State Animation){UniqueID=18628, TimeStep=1/300}
      mask prompts: UniqueID "Auto-Assigned: Unique ID"; TimeStep "Auto-Assigned: Upload Period [s]"
      mask help: The Human Animation port allows the human to walk, run or bend
      mask Help: eval('openHelp(239)')
      mask Display: image(imread('HumanAnimated.jpg'))
  wires:
  ANIM_Child_RegularAni_2/1 -> Actuator/1

== system World_01_Base_Map_cs/ANIM_Female_RegularAni_1 ==
  ANIM_Female_RegularAni_1 : Inport  Tag=inport/AnimationOutport  OutDataTypeStr=Bus: PRESCAN_ANIMACTUATORDATA  PortDimensions=1  SampleTime=1/300  BusOutputAsStruct=on
  Actuator : S-Function  FunctionName=sfun_AnimActuator  Parameters=UniqueID, TimeStep  SFunctionDeploymentMode=off  EnableBusSupport=off  mask(PreScan Sink Block: State Animation){UniqueID=18631, TimeStep=1/300}
      mask prompts: UniqueID "Auto-Assigned: Unique ID"; TimeStep "Auto-Assigned: Upload Period [s]"
      mask help: The Human Animation port allows the human to walk, run or bend
      mask Help: eval('openHelp(239)')
      mask Display: image(imread('HumanAnimated.jpg'))
  wires:
  ANIM_Female_RegularAni_1/1 -> Actuator/1

== system World_01_Base_Map_cs/ANIM_Male_RegularAni_1 ==
  ANIM_Male_RegularAni_1 : Inport  Tag=inport/AnimationOutport  OutDataTypeStr=Bus: PRESCAN_ANIMACTUATORDATA  PortDimensions=1  SampleTime=1/300  BusOutputAsStruct=on
  Actuator : S-Function  FunctionName=sfun_AnimActuator  Parameters=UniqueID, TimeStep  SFunctionDeploymentMode=off  EnableBusSupport=off  mask(PreScan Sink Block: State Animation){UniqueID=18634, TimeStep=1/300}
      mask prompts: UniqueID "Auto-Assigned: Unique ID"; TimeStep "Auto-Assigned: Upload Period [s]"
      mask help: The Human Animation port allows the human to walk, run or bend
      mask Help: eval('openHelp(239)')
      mask Display: image(imread('HumanAnimated.jpg'))
  wires:
  ANIM_Male_RegularAni_1/1 -> Actuator/1

== system World_01_Base_Map_cs/ANIM_Male_RegularAni_2 ==
  ANIM_Male_RegularAni_2 : Inport  Tag=inport/AnimationOutport  OutDataTypeStr=Bus: PRESCAN_ANIMACTUATORDATA  PortDimensions=1  SampleTime=1/300  BusOutputAsStruct=on
  Actuator : S-Function  FunctionName=sfun_AnimActuator  Parameters=UniqueID, TimeStep  SFunctionDeploymentMode=off  EnableBusSupport=off  mask(PreScan Sink Block: State Animation){UniqueID=18853, TimeStep=1/300}
      mask prompts: UniqueID "Auto-Assigned: Unique ID"; TimeStep "Auto-Assigned: Upload Period [s]"
      mask help: The Human Animation port allows the human to walk, run or bend
      mask Help: eval('openHelp(239)')
      mask Display: image(imread('HumanAnimated.jpg'))
  wires:
  ANIM_Male_RegularAni_2/1 -> Actuator/1

== system World_01_Base_Map_cs/Audi_A8_Sedan_1 ==
  SELF_Audi_A8_Sedan_1 : Inport  Tag=inport/SelfPort  OutDataTypeStr=Bus: PRESCAN_SELFSENSORDATA  PortDimensions=1  SampleTime=1/300  BusOutputAsStruct=on
  Car_Pos_and_Orient : Subsystem
  Path : S-Function  Tag=Path  LoadFcn=load('PrescanMotionData.mat')  FunctionName=sfun_Path  Parameters=uniqueID, pathUniqueID, timestep  SFunctionDeploymentMode=off  EnableBusSupport=off  mask(Path){uniqueID=18645, pathUniqueID=18644, timestep=1/300}
      mask prompts: uniqueID "Object Unique ID"; pathUniqueID "Path Unique ID"; timestep "MATLAB timestep:"
      mask help:
      | The path block outputs the position along a given trajectory.
      |
      | For more information, please click Help.
      mask Help: eval('openHelp(312)')
      mask Display: image(imread('Path.png'))
  SELF_Demux : Subsystem  Tag=demux/SelfPort  mask(PreScan Demux Block:){}
      mask help:
      | The SELF port shows (state) information of the actor itself. The outputs are position in the experiment's axis system and the GPS coordinates, and the object's absolute velocity and compass heading.
      |
      | For more information, please click Help.
      settings: DeleteFcn=PreScanBlockDeleteFcn;
      mask Help: eval('openHelp(462)')
      mask Display:
      | port_label('output',1,'x [m]')
      | port_label('output',2,'y [m]')
      | port_label('output',3,'z [m]','texmode','on')
      | port_label('output',4,'Rotx [deg]','texmode','on')
      | port_label('output',5,'Roty [deg]','texmode','on')
      | port_label('output',6,'Rotz [deg]','texmode','on')
      | port_label('output',7,'GPS lat [deg]','texmode','on')
      | port_label('output',8,'GPS long [deg]','texmode','on')
      | port_label('output',9,'GPS alt [m]','texmode','on')
      | port_label('output',10,'Velocity [m/s]')
      | port_label('output',11,'Heading [deg]')
      | port_label('output',12,'Yaw rate [deg/s]')
  STATE_Audi_A8_Sedan_1_rc : RateTransition  Tag=mux_rc/StatePort  OutPortSampleTimeOpt=Inherit
  SpeedProfile : S-Function  Tag=SpeedProfile  LoadFcn=load('PrescanMotionData.mat')  FunctionName=sfun_SpeedProfile  Parameters=speedProfileUniqueID, timestep  SFunctionDeploymentMode=off  EnableBusSupport=off  mask(SpeedProfile){speedProfileUniqueID=18646, timestep=1/300}
      mask prompts: speedProfileUniqueID "Speed Profile Unique ID"; timestep "MATLAB timestep:"
      mask help:
      | The speed profile block outputs the travelled distance, velocities and acceleration along a given path.
      |
      | For more information, please click Help.
      mask Help: eval('openHelp(312)')
      mask Display: image(imread('SpeedProfile.png'))
  Terminator_{1..6} (6 alike) : Terminator
  message_creator : Subsystem
  STATE_Audi_A8_Sedan_1_bus : Outport  Tag=outport/StatePort  OutDataTypeStr=Bus: PRESCAN_STATEACTUATORDATA  PortDimensions=1  SampleTime=1/300
  SafetyPlannerLoc : Outport  Port=2
  wires:
  Car_Pos_and_Orient/1(Out1) -> message_creator/1(In1)
  message_creator/1(Out1) -> SafetyPlannerLoc/1
  SELF_Demux/1(x [m]) -> Car_Pos_and_Orient/1(In1)
  SELF_Demux/2(y [m]) -> Car_Pos_and_Orient/2(In2)
  SELF_Demux/3(z [m]) -> Car_Pos_and_Orient/3(In3)
  SELF_Demux/4(rotx [deg]) -> Car_Pos_and_Orient/4(In4)
  SELF_Demux/5(roty [deg]) -> Car_Pos_and_Orient/5(In5)
  SELF_Demux/6(rotz [deg]) -> Car_Pos_and_Orient/6(In6)
  STATE_Audi_A8_Sedan_1_rc/1 -> STATE_Audi_A8_Sedan_1_bus/1
  SpeedProfile/1 -> Path/1
  Path/1 -> STATE_Audi_A8_Sedan_1_rc/1
  SELF_Audi_A8_Sedan_1/1 -> SELF_Demux/1(SELF)
  SELF_Demux/7(GPS lat [deg]) -> Terminator_1/1
  SELF_Demux/8(GPS long [deg]) -> Terminator_2/1
  SELF_Demux/9(GPS alt [m]) -> Terminator_3/1
  SELF_Demux/10(velocity [m/s]) -> Terminator_4/1
  SELF_Demux/11(heading [deg]) -> Terminator_5/1
  SELF_Demux/12(yaw rate [deg/s]) -> Terminator_6/1
